simulink model "AFE_PontHPV3"  (R2013b)
settings: Solver=FixedStepDiscrete  SolverMode=SingleTasking  StartTime=0.0  StopTime=inf  FixedStep=Tpas  MinStep=Tpas  RelTol=1e-3
values from neighbouring files (symbols this model uses):
  Cbus = 300e-3    (= 0.3)    [AFE_FV_Params.m]    (also in AFE_PontHPV2.m; AFEsimpleparacph1REgVPV2.m; initAFE_PontHPV3.m)
  fmod = 1e3    (= 1000)    [AFE_PontHPV2.m]    (also in initAFE_PontHPV3.m)
  Freq = 50    [AFE_2L_RC_param_DT1.m]    (also in AFE_FV_Params.m; AFE_PontHPV2.m; AFEsimplepara.m; AFEsimpleparaDT1.m)
  hys = 100    [AFE_2L_RC_param_DT1.m]    (also in AFE_FV_Params.m = 150; AFE_PontHPV2.m = 150; AFEsimplepara.m = 0.1; AFEsimpleparaDT1.m)
  I = (P+Numd(2)/Dend(1))/Ts    [AFE_2L_RC_param_DT1.m]    (also in AFE_PontHPV2.m; AFEsimpleparaDT1.m; AFEsimpleparaPV2.m; initAFE_PontHPV3.m)
  Iv = (Pv+Numdv(2)/Dendv(1))/Tsv    [AFE_PontHPV2.m]    (also in AFEsimpleparacph1REgVPV2.m; initAFE_PontHPV3.m)
  Kac = 1/(Vac*sqrt(2/3))    [AFE_FV_Params.m]    (also in AFE_PontHPV2.m; AFEsimpleparacph1REgVPV2.m; initAFE_PontHPV3.m)
  KLP = NLPripd(2)    [AFE_PontHPV2.m]    (also in initAFE_PontHPV3.m)
  L = .1    (= 0.1)    [AFE_PontHPV2.m]    (also in initAFE_PontHPV3.m)
  Lac = 8.1487e-04    (= 0.00081487)    [AFE_2L_RC_param_DT1.m]    (also in AFE_FV_Params.m; AFE_PontHPV2.m; AFEsimplepara.m = 0.002; AFEsimpleparaDT1.m)
  P = Numd(1)/Dend(1)    [AFE_2L_RC_param_DT1.m]    (also in AFE_PontHPV2.m; AFEsimpleparaDT1.m; AFEsimpleparaPV2.m; initAFE_PontHPV3.m)
  Pv = Numdv(1)/Dendv(1)    [AFE_PontHPV2.m]    (also in AFEsimpleparacph1REgVPV2.m; initAFE_PontHPV3.m)
  R = 9.26    [AFE_2L_RC_param_DT1.m]    (also in AFE_PontHPV2.m = 0.28; AFEsimpleparaDT1.m; AFEsimpleparaPV2.m; initAFE_PontHPV3.m = 0.28)
  Rac = 2.5    [AFEsimplepara.m]
  Sat = .95    (= 0.95)    [AFE_PontHPV2.m]    (also in AFEsimpleparaDT1.m = 5000; AFEsimpleparaPV2.m = 5000; initAFE_PontHPV3.m)
  Satv = 5000    [AFE_PontHPV2.m]    (also in AFEsimpleparacph1REgVPV2.m; initAFE_PontHPV3.m = 1500)
  TLP = DLPripd(2)    [AFE_PontHPV2.m]    (also in initAFE_PontHPV3.m)
  Tpas = 5e-5    (= 5e-05)    [AFE_2L_RC_param_DT1.m]    (also in AFE_FV_Params.m; AFE_PontHPV2.m = 3e-06; AFEsimplepara.m = 1e-05; AFEsimpleparaDT1.m)
  Tstep = Tpas    (= 3e-06)    [AFE_PontHPV2.m]    (also in initAFE_PontHPV3.m)
  Vac = 2000    [AFE_2L_RC_param_DT1.m]    (also in AFE_FV_Params.m; AFE_PontHPV2.m; AFEsimplepara.m; AFEsimpleparaDT1.m)
libraries: powerlib x28, simulink x6, powerlib_meascontrol x6
settings Model: Creator=LiberT  LastModifiedBy=philippe
settings DataIOCC: SignalLoggingSaveFormat=ModelDataLogs
settings OptimizationCC: ExpressionDepthLimit=2147483647
settings DebuggingCC: MultiTaskDSMMsg=warning  MultiTaskCondExecSysMsg=none  FcnCallInpInsideContextMsg=EnableAllAsWarning  UnconnectedInputMsg=none  UnconnectedOutputMsg=none  UnconnectedLineMsg=none  StateNameClashWarn=warning  StrictBusMsg=None
settings RTWCC: IncludeERTFirstTime=on

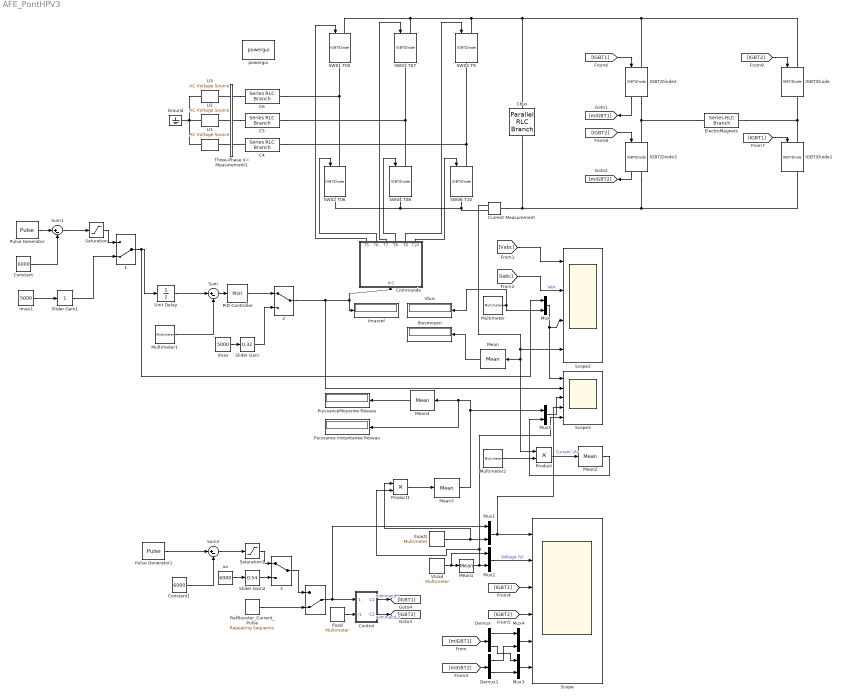
== system AFE_PontHPV3 ==
  " " : ManualSwitch  CurrentSetting=0
  " 1" : ManualSwitch  CurrentSetting=0
  " 2" : ManualSwitch
  " 3" : ManualSwitch
  C4 : powerlib/Elements/Series RLC Branch  LConnTagsString=__new0  RConnTagsString=__new0  BranchType=L  Resistance=Rac  Inductance=Lac  SetiL0=off  InitialCurrent=0  Capacitance=300e-3  Setx0=off  InitialVoltage=0  Measurements=None
  C5 : powerlib/Elements/Series RLC Branch  LConnTagsString=__new0  RConnTagsString=__new0  BranchType=L  Resistance=Rac  Inductance=Lac  SetiL0=off  InitialCurrent=0  Capacitance=300e-3  Setx0=off  InitialVoltage=0  Measurements=None
  C6 : powerlib/Elements/Series RLC Branch  LConnTagsString=__new0  RConnTagsString=__new0  BranchType=L  Resistance=Rac  Inductance=Lac  SetiL0=off  InitialCurrent=0  Capacitance=300e-3  Setx0=off  InitialVoltage=0  Measurements=None
  Cbus : powerlib/Elements/Parallel RLC Branch  LConnTagsString=a  RConnTagsString=__new0  BranchType=C  Resistance=inf  Inductance=inf  SetiL0=off  InitialCurrent=0  Capacitance=Cbus  Setx0=on  InitialVoltage=Vdc  Measurements=Branch voltage
  Commande : Subsystem
  Constant : Constant  Value=6000
  Constant1 : Constant  Value=6000
  Control : Subsystem  TreatAsAtomicUnit=on
      settings: MinAlgLoopOccurrences=on
  Current Measurement : powerlib/Measurements/Current Measurement  PhasorSimulation=off  OutputType=Complex  PSBequivalent=0
  Demux : Demux  Outputs=2
  Demux1 : Demux  Outputs=2
  "ElectroMagnets " : powerlib/Elements/Series RLC Branch  LConnTagsString=__new0  RConnTagsString=__new0  BranchType=RL  Resistance=R  Inductance=L  SetiL0=off  InitialCurrent=0  Capacitance=1e-6  Setx0=off  InitialVoltage=0  Measurements=Branch voltage and current
  Ground : powerlib/Elements/Ground  LConnTagsString=a
  IGBT/Diode{,1..3} (4 alike) : powerlib/Power Electronics/IGBT//Diode  Ron=1e-3  Rs=1e5  Cs=inf  Measurements=on
  Ibusmoyen : Display
  Iload : powerlib/Measurements/Multimeter  PhasorSimulation=off  OutputType=Complex  sel=6  L=6  Gain=1  yselected={'Ib: ElectroMagnets '};  PSBOutputType=1  PSBequivalent=0  AxesSetting=[0,0.1,-100,100]  Display=0  SavedBlockNames=-11
  Iload1 : powerlib/Measurements/Multimeter  PhasorSimulation=off  OutputType=Complex  sel=6  L=6  Gain=1  yselected={'Ib: ElectroMagnets '};  PSBOutputType=1  PSBequivalent=0  AxesSetting=[0,0.1,-100,100]  Display=0  SavedBlockNames=-11
  Imax : Constant  Value=5000
  Imax1 : Constant  Value=5000
  Imaxref : Display
  Mean : powerlib_meascontrol/Measurements/Mean  Freq=60  Vinit=0  Ts=Tpas
  Mean1 : powerlib_meascontrol/Measurements/Mean  Freq=fmod  Vinit=0  Ts=Tpas
  Mean2 : powerlib_meascontrol/Measurements/Mean  Freq=fmod  Vinit=0  Ts=Tpas
  Mean3 : powerlib_meascontrol/Measurements/Mean  Freq=fmod/2  Vinit=0  Ts=Tpas
  Mean4 : powerlib_meascontrol/Measurements/Mean  Freq=1/900e-3  Vinit=0  Ts=Tpas
  Multimeter : powerlib/Measurements/Multimeter  PhasorSimulation=off  OutputType=Complex  sel=2  L=6  Gain=1  yselected={'Ub: Cbus'};  PSBOutputType=1  PSBequivalent=0  AxesSetting=[0,0.1,-100,100]  Display=0  SavedBlockNames=-11
  Multimeter1 : powerlib/Measurements/Multimeter  PhasorSimulation=off  OutputType=Complex  sel=2  L=6  Gain=1  yselected={'Ub: Cbus'};  PSBOutputType=1  PSBequivalent=0  AxesSetting=[0,0.1,-100,100]  Display=0  SavedBlockNames=-11
  Multimeter2 : powerlib/Measurements/Multimeter  PhasorSimulation=off  OutputType=Complex  sel=2  L=6  Gain=1  yselected={'Ub: Cbus'};  PSBOutputType=1  PSBequivalent=0  AxesSetting=[0,0.1,-100,100]  Display=0  SavedBlockNames=-11
  Mux{,1..5} (6 alike) : Mux  Inputs=2
  PID Controller : simulink/Continuous/PID Controller  Controller=PI  TimeDomain=Discrete-time  SampleTime=Tpas  IntegratorMethod=Forward Euler  FilterMethod=Forward Euler  Form=Parallel  P=Pv  I=Iv  D=0  N=100  InitialConditionSource=internal  InitialConditionForIntegrator=0  InitialConditionForFilter=0  ExternalReset=none  LimitOutput=on  UpperSaturationLimit=Satv  LowerSaturationLimit=-Satv  LinearizeAsGain=on  AntiWindupMode=clamping  Kb=1  TrackingMode=off  Kt=1  PParamMin=[]  PParamMax=[]  IParamMin=[]  IParamMax=[]  DParamMin=[]  DParamMax=[]  NParamMin=[]  NParamMax=[]  KbParamMin=[]  KbParamMax=[]  KtParamMin=[]  KtParamMax=[]  POutMin=[]  POutMax=[]  IOutMin=[]  IOutMax=[]  DOutMin=[]  DOutMax=[]  NOutMin=[]  NOutMax=[]  KbOutMin=[]  KbOutMax=[]  KtOutMin=[]  KtOutMax=[]  IntegratorOutMin=[]  IntegratorOutMax=[]  FilterOutMin=[]  FilterOutMax=[]  SumOutMin=[]  SumOutMax=[]  SumI1OutMin=[]  SumI1OutMax=[]  SumI2OutMin=[]  SumI2OutMax=[]  SumI3OutMin=[]  SumI3OutMax=[]  SumDOutMin=[]  SumDOutMax=[]  SaturationOutMin=[]  SaturationOutMax=[]  IntegratorContinuousStateAttributes=''  IntegratorStateMustResolveToSignalObject=off  IntegratorRTWStateStorageClass=Auto  FilterContinuousStateAttributes=''  FilterStateMustResolveToSignalObject=off  FilterRTWStateStorageClass=Auto
  Product : Product
  Product1 : Product
  "Puissance instantanée Réseau " : Display
  PuissanceMoyenne Réseau : Display
  Pulse Generator : DiscretePulseGenerator  Amplitude=12000  Period=floor(.2/Tpas)  PulseWidth=floor(.2/2/Tpas)  SampleTime=Tpas
  Pulse Generator1 : DiscretePulseGenerator  Amplitude=12000  Period=floor(.6/Tpas)  PulseWidth=floor(.6/2/Tpas)  SampleTime=Tpas
  "RefBooster_Current_Pulse " : simulink/Sources/Repeating Sequence  rep_seq_t=[0 100e-3 100.1e-3 475e-3 550e-3 708.4e-3 900e-3]  rep_seq_y=[0 0 250 6000 6000 250 250]
  SW01 T05 : powerlib/Power Electronics/IGBT//Diode  Ron=1e-3  Rs=1e5  Cs=Tpas  Measurements=off
  SW02 T06 : powerlib/Power Electronics/IGBT//Diode  Ron=1e-3  Rs=1e5  Cs=Tpas  Measurements=off
  SW03 T07 : powerlib/Power Electronics/IGBT//Diode  Ron=1e-3  Rs=1e5  Cs=Tpas  Measurements=off
  SW04 T08 : powerlib/Power Electronics/IGBT//Diode  Ron=1e-3  Rs=1e5  Cs=Tpas  Measurements=off
  SW05 T9 : powerlib/Power Electronics/IGBT//Diode  Ron=1e-3  Rs=1e5  Cs=Tpas  Measurements=off
  SW06 T10 : powerlib/Power Electronics/IGBT//Diode  Ron=1e-3  Rs=1e5  Cs=Tpas  Measurements=off
  Saturation : Saturate  UpperLimit=5200  LowerLimit=5100
  Saturation1 : Saturate  UpperLimit=5000  LowerLimit=2000
  Scope : Scope  NumInputPorts=6
      settings: TimeRange=2  YMin=-7000~-12500~-0.1~-0.1~-7000~-6000  YMax=7000~7500~1.1~1.1~7000~6000  SaveName=ScopeData2
  Scope2 : Scope  NumInputPorts=4
      settings: TickLabels=on  TimeRange=0.04  YMin=-1750~-2000~0~-2000  YMax=1750~2000~5500~2000
  Scope3 : Scope  NumInputPorts=5
      settings: TickLabels=on  TimeRange=2  YMin=0~-3000~-20000000~-100~-5500  YMax=5500~3000~20000000~6500~5500
  Slider Gain : simulink/Math Operations/Slider Gain  low=0  gain=0.32  high=1
  Slider Gain1 : simulink/Math Operations/Slider Gain  low=0  gain=1  high=1
  Slider Gain2 : simulink/Math Operations/Slider Gain  low=0  gain=0.54  high=1
  Sum : Sum  Inputs=|+-
  Sum1 : Sum  Inputs=|+-
  Sum2 : Sum  Inputs=|+-
  Three-Phase V-I Measurement1 : powerlib/Measurements/Three-Phase V-I Measurement  VoltageMeasurement=phase-to-ground  SetLabelV=on  LabelV=Vabc  Vpu=off  VpuLL=off  CurrentMeasurement=yes  SetLabelI=on  LabelI=Iabc  Ipu=off  Pbase=100e6  Vbase=500e3  OutputType=Complex  PhasorSimulation=off  PSBequivalent=0
  U1 : powerlib/Electrical Sources/AC Voltage Source  Amplitude=Vac*sqrt(2/3)  Phase=240  Frequency=Freq  SampleTime=0  Measurements=Voltage
  U2 : powerlib/Electrical Sources/AC Voltage Source  Amplitude=Vac*sqrt(2/3)  Phase=120  Frequency=Freq  SampleTime=0  Measurements=Voltage
  U3 : powerlib/Electrical Sources/AC Voltage Source  Amplitude=Vac*sqrt(2/3)  Phase=0  Frequency=Freq  SampleTime=0  Measurements=Voltage
  Unit Delay : UnitDelay  SampleTime=-1
  Vbus : Display
  Vload : powerlib/Measurements/Multimeter  PhasorSimulation=off  OutputType=Complex  sel=1  L=6  Gain=1  yselected={'Ub: ElectroMagnets '};  PSBOutputType=1  PSBequivalent=0  AxesSetting=[0,0.1,-100,100]  Display=0  SavedBlockNames=-11
  powergui : powerlib/powergui  Priority=1  SimulationMode=Discrete  SolverType=Tustin  SampleTime=Tpas  frequency=60  SPID=off  DisableSnubberDevices=off  DisableRonSwitches=off  DisableVfSwitches=off  SwTol=0  Interpol=off  DisplayEquations=off  frequencyindice=50  Pbase=100e6  ErrMax=1e-4  Iterations=50  UnitsV=kV  UnitsW=MW  FunctionMessages=off  echomessages=off  HookPort=off  EnableUseOfTLC=off  x0status=blocks  RestoreLinks=warning  ResistiveCurrentMeasurement=off  Frange=[0:2:500]  Ylog=off  Xlog=on  ShowGrid=off  save=off  variable=ZData  structure=ScopeData1  ZoomFFT=off  StartTime=18  cycles=100  DisplayStyle=1  fundamental=50  FreqAxis=off  MaxFrequency=2000  frequencyindicesteady=1  RmsSteady=1  display=off  Ts=0  methode=off
  uo : Constant  Value=6000
  wires:
  Commande/1(T5) -> SW01 T05/1
  Commande/2(T6) -> SW02 T06/1
  Commande/4(T8) -> SW04 T08/1
  Commande/3(T7) -> SW03 T07/1
  Commande/6(T10) -> SW06 T10/1
  Commande/5(T9) -> SW05 T9/1
  [Vabc] -> Scope2/1
  Current Measurement/1 -> Scope2/4, Product/1, Mean/1
  Multimeter/1 -> Vbus/1, Mux/2
  Mean/1 -> Ibusmoyen/1
  " 2"/1 -> Scope3/2, Commande/1(In1), Imaxref/1
  Multimeter1/1 -> Sum/2
  Sum/1 -> PID Controller/1
  Unit Delay/1 -> Sum/1
  Imax1/1 -> Slider Gain1/1
  " 1"/1 -> Mux/1, Unit Delay/1
  Saturation/1 -> " 1"/1
  Sum1/1 -> Saturation/1
  Pulse Generator/1 -> Sum1/1
  Constant/1 -> Sum1/2
  Slider Gain1/1 -> " 1"/2
  PID Controller/1 -> " 2"/1
  Imax/1 -> Slider Gain/1
  Slider Gain/1 -> " 2"/2
  Mux/1 -> Scope2/3, Scope3/1
  [Iabc] -> Scope2/2  "Iabc"
  Mux1/1 -> Scope3/4, Scope/1  "Current (A)"
  Mux2/1 -> Scope/2  "Voltage (V)"
  IGBT/Diode2/1 -> [mIGBT1]
  IGBT/Diode3/1 -> [mIGBT2]
  uo/1 -> Slider Gain2/1
  "RefBooster_Current_Pulse "/1 -> " "/2
  " 3"/1 -> " "/1
  Slider Gain2/1 -> " 3"/2
  Saturation1/1 -> " 3"/1
  " "/1 -> Control/1(Iref), Mux1/1
  Iload1/1 -> Product1/1, Mux1/2
  Iload/1 -> Control/2(IL)
  [mIGBT1] -> Demux/1
  Mean1/1 -> Product1/2, Scope3/5, Mux2/2
  Vload/1 -> Mux2/1, Mean1/1
  [IGBT1] -> IGBT/Diode2/1
  Control/1(C1) -> [IGBT1]  "Command 1"
  [IGBT1] -> IGBT/Diode1/1
  Control/2(C2) -> [IGBT2]  "Command 2"
  [IGBT2] -> IGBT/Diode3/1
  [IGBT2] -> IGBT/Diode/1
  [mIGBT2] -> Demux1/1
  [IGBT1] -> Scope/3
  Mux3/1 -> Scope/6
  Mux4/1 -> Scope/5
  [IGBT2] -> Scope/4
  Sum2/1 -> Saturation1/1
  Pulse Generator1/1 -> Sum2/1
  Constant1/1 -> Sum2/2
  Demux/1 -> Mux4/1
  Demux1/1 -> Mux4/2
  Demux/2 -> Mux3/1
  Demux1/2 -> Mux3/2
  Multimeter2/1 -> Product/2
  Product/1 -> Mean2/1
  Product1/1 -> Mean3/1
  Mux5/1 -> Scope3/3
  Mean2/1 -> Mux5/2
  Mean3/1 -> "Puissance instantanée Réseau "/1, Mean4/1, Mux5/1
  Mean4/1 -> PuissanceMoyenne Réseau/1
  connections:
  SW02 T06/RConn1 -- Current Measurement/RConn1 -- SW06 T10/RConn1 -- SW04 T08/RConn1
  IGBT/Diode2/LConn1 -- IGBT/Diode/LConn1 -- SW01 T05/LConn1 -- SW03 T07/LConn1 -- SW05 T9/LConn1 -- Cbus/LConn1
  SW02 T06/LConn1 -- C6/LConn1 -- SW01 T05/RConn1
  SW06 T10/LConn1 -- C4/LConn1 -- SW05 T9/RConn1
  SW04 T08/LConn1 -- SW03 T07/RConn1 -- C5/LConn1
  U2/LConn1 -- U1/LConn1 -- Ground/LConn1 -- U3/LConn1
  Three-Phase V-I Measurement1/LConn1 -- C6/RConn1
  Three-Phase V-I Measurement1/RConn1 -- U3/RConn1
  U2/RConn1 -- Three-Phase V-I Measurement1/RConn2
  Three-Phase V-I Measurement1/LConn2 -- C5/RConn1
  C4/RConn1 -- Three-Phase V-I Measurement1/LConn3
  U1/RConn1 -- Three-Phase V-I Measurement1/RConn3
  IGBT/Diode3/RConn1 -- Cbus/RConn1 -- Current Measurement/LConn1 -- IGBT/Diode1/RConn1
  "ElectroMagnets "/LConn1 -- IGBT/Diode2/RConn1 -- IGBT/Diode3/LConn1
  IGBT/Diode/RConn1 -- "ElectroMagnets "/RConn1 -- IGBT/Diode1/LConn1

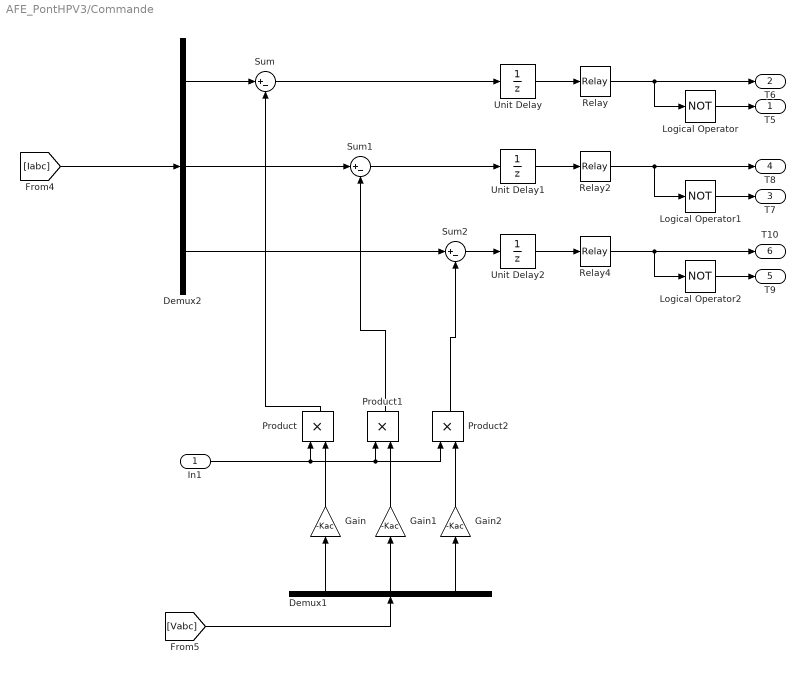
== system AFE_PontHPV3/Commande ==
  In1 : Inport
  Demux1 : Demux  Outputs=3
  Demux2 : Demux  Outputs=3
  Gain : Gain  Gain=-Kac
  Gain1 : Gain  Gain=-Kac
  Gain2 : Gain  Gain=-Kac
  Logical Operator : Logic  Operator=NOT  AllPortsSameDT=off
  Logical Operator1 : Logic  Operator=NOT  AllPortsSameDT=off
  Logical Operator2 : Logic  Operator=NOT  AllPortsSameDT=off
  Product : Product
  Product1 : Product
  Product2 : Product
  Relay : Relay  OnSwitchValue=hys  OffSwitchValue=-hys
  Relay2 : Relay  OnSwitchValue=hys  OffSwitchValue=-hys
  Relay4 : Relay  OnSwitchValue=hys  OffSwitchValue=-hys
  Sum : Sum  Inputs=|+-
  Sum1 : Sum  Inputs=|+-
  Sum2 : Sum  Inputs=|+-
  Unit Delay : UnitDelay  SampleTime=-1
  Unit Delay1 : UnitDelay  SampleTime=-1
  Unit Delay2 : UnitDelay  SampleTime=-1
  T5 : Outport
  T6 : Outport  Port=2
  T7 : Outport  Port=3
  T8 : Outport  Port=4
  T9 : Outport  Port=5
  T10 : Outport  Port=6
  wires:
  Demux2/1 -> Sum/1
  Demux2/2 -> Sum1/1
  Demux2/3 -> Sum2/1
  Sum/1 -> Unit Delay/1
  Sum1/1 -> Unit Delay1/1
  Sum2/1 -> Unit Delay2/1
  Unit Delay/1 -> Relay/1
  Unit Delay1/1 -> Relay2/1
  Unit Delay2/1 -> Relay4/1
  Logical Operator/1 -> T5/1
  Logical Operator1/1 -> T7/1
  Logical Operator2/1 -> T9/1
  Relay/1 -> T6/1, Logical Operator/1
  Relay2/1 -> T8/1, Logical Operator1/1
  Relay4/1 -> T10/1, Logical Operator2/1
  [Iabc] -> Demux2/1
  [Vabc] -> Demux1/1
  Demux1/1 -> Gain/1
  Demux1/2 -> Gain1/1
  Demux1/3 -> Gain2/1
  Gain/1 -> Product/2
  Gain1/1 -> Product1/2
  Gain2/1 -> Product2/2
  In1/1 -> Product2/1, Product1/1, Product/1
  Product/1 -> Sum/2
  Product1/1 -> Sum1/2
  Product2/1 -> Sum2/2

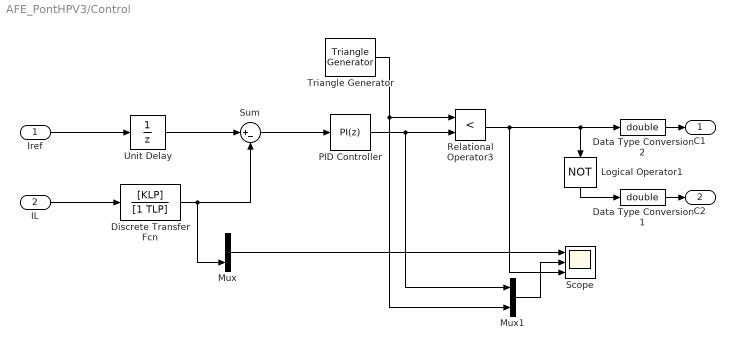
== system AFE_PontHPV3/Control ==
  Iref : Inport
  IL : Inport  Port=2
  Data Type Conversion1 : DataTypeConversion  OutDataTypeStr=double
  Data Type Conversion2 : DataTypeConversion  OutDataTypeStr=double
  Discrete Transfer Fcn : DiscreteTransferFcn  Numerator=[KLP]  Denominator=[1 TLP]
  Logical Operator1 : Logic  Operator=NOT  AllPortsSameDT=off  OutDataTypeStr=boolean
  Mux : Mux  Inputs=2
  Mux1 : Mux  Inputs=2
  PID Controller : simulink/Continuous/PID Controller  Controller=PI  TimeDomain=Discrete-time  SampleTime=Tstep  IntegratorMethod=Forward Euler  FilterMethod=Forward Euler  Form=Parallel  P=P  I=I  D=0  N=100  InitialConditionSource=internal  InitialConditionForIntegrator=0  InitialConditionForFilter=0  ExternalReset=none  LimitOutput=on  UpperSaturationLimit=Sat  LowerSaturationLimit=-Sat  LinearizeAsGain=on  AntiWindupMode=clamping  Kb=1  TrackingMode=off  Kt=1  PParamMin=[]  PParamMax=[]  IParamMin=[]  IParamMax=[]  DParamMin=[]  DParamMax=[]  NParamMin=[]  NParamMax=[]  KbParamMin=[]  KbParamMax=[]  KtParamMin=[]  KtParamMax=[]  POutMin=[]  POutMax=[]  IOutMin=[]  IOutMax=[]  DOutMin=[]  DOutMax=[]  NOutMin=[]  NOutMax=[]  KbOutMin=[]  KbOutMax=[]  KtOutMin=[]  KtOutMax=[]  IntegratorOutMin=[]  IntegratorOutMax=[]  FilterOutMin=[]  FilterOutMax=[]  SumOutMin=[]  SumOutMax=[]  SumI1OutMin=[]  SumI1OutMax=[]  SumI2OutMin=[]  SumI2OutMax=[]  SumI3OutMin=[]  SumI3OutMax=[]  SumDOutMin=[]  SumDOutMax=[]  SaturationOutMin=[]  SaturationOutMax=[]  IntegratorContinuousStateAttributes=''  IntegratorStateMustResolveToSignalObject=off  IntegratorRTWStateStorageClass=Auto  FilterContinuousStateAttributes=''  FilterStateMustResolveToSignalObject=off  FilterRTWStateStorageClass=Auto
  Relational Operator3 : RelationalOperator  Operator=<  OutDataTypeStr=boolean
  Scope : Scope  NumInputPorts=3
      settings: YMin=0~-1~-5  YMax=6500~1~5  SaveName=ScopeData3
  Sum : Sum  Inputs=|+-
  Triangle Generator : powerlib_meascontrol/Pulse & Signal Generators/Triangle Generator  Freq=fmod  Phase=180  Ts=Tstep
  Unit Delay : UnitDelay  SampleTime=-1
  C1 : Outport
  C2 : Outport  Port=2
  wires:
  Triangle Generator/1 -> Mux1/2, Relational Operator3/1
  Relational Operator3/1 -> Scope/3, Logical Operator1/1, Data Type Conversion2/1
  Data Type Conversion2/1 -> C1/1
  Logical Operator1/1 -> Data Type Conversion1/1
  Data Type Conversion1/1 -> C2/1
  Mux/1 -> Scope/1
  Mux1/1 -> Scope/2
  PID Controller/1 -> Relational Operator3/2, Mux1/1
  Discrete Transfer Fcn/1 -> Mux/2, Sum/2
  Sum/1 -> PID Controller/1
  IL/1 -> Discrete Transfer Fcn/1
  Iref/1 -> Unit Delay/1
  Unit Delay/1 -> Sum/1
